simulink model "Teensy_Model"  (R2025b)
settings: Solver=FixedStepAuto  StartTime=0.0  StopTime=Inf  FixedStep=ts  RelTol=1e-3  EnableMultiTasking=on
model workspace (MAT data in the model file):
  Footcontrol = Simulink.Parameter
  Footcontrol.Value = 0
  Footcontrol.Complexity = 'real'
  Footcontrol.Dimensions = [1 1]
  Footcontrol.Description = 'Footcontrol'
  Footcontrol.DataType = 'uint8'
  GPIO_0 = Simulink.Parameter
  GPIO_0.Value = 0
  GPIO_0.Complexity = 'real'
  GPIO_0.Dimensions = [1 1]
  GPIO_0.Description = 'GPIO_0'
  GPIO_0.DataType = 'boolean'
  GPIO_1 = Simulink.Parameter
  GPIO_1.Value = 0
  GPIO_1.Complexity = 'real'
  GPIO_1.Dimensions = [1 1]
  GPIO_1.Description = 'GPIO_1'
  GPIO_1.DataType = 'boolean'
  GPIO_2 = Simulink.Parameter
  GPIO_2.Value = 0
  GPIO_2.Complexity = 'real'
  GPIO_2.Dimensions = [1 1]
  GPIO_2.Description = 'GPIO_2'
  GPIO_2.DataType = 'boolean'
  GPIO_3 = Simulink.Signal
  GPIO_3.Dimensions = -1
  GPIO_3.DimensionsMode = 'auto'
  GPIO_3.Complexity = 'real'
  GPIO_3.SampleTime = -1
  GPIO_3.SamplingMode = 'auto'
  GPIO_3.Description = 'GPIO_3'
  GPIO_3.DataType = 'uint16'
  GPIO_4 = Simulink.Signal
  GPIO_4.Dimensions = -1
  GPIO_4.DimensionsMode = 'auto'
  GPIO_4.Complexity = 'real'
  GPIO_4.SampleTime = -1
  GPIO_4.SamplingMode = 'auto'
  GPIO_4.Description = 'GPIO_4'
  GPIO_4.DataType = 'uint16'
  GPIO_5 = Simulink.Signal
  GPIO_5.Dimensions = -1
  GPIO_5.DimensionsMode = 'auto'
  GPIO_5.Complexity = 'real'
  GPIO_5.SampleTime = -1
  GPIO_5.SamplingMode = 'auto'
  GPIO_5.Description = 'GPIO_5'
  GPIO_5.DataType = 'uint16'
  MD_Current = Simulink.Signal
  MD_Current.Dimensions = -1
  MD_Current.DimensionsMode = 'auto'
  MD_Current.Complexity = 'real'
  MD_Current.SampleTime = -1
  MD_Current.SamplingMode = 'auto'
  MD_Current.Description = 'MD_Current'
  MD_Current.DataType = 'uint16'
  Motor_Enable = Simulink.Parameter
  Motor_Enable.Value = 0
  Motor_Enable.Complexity = 'real'
  Motor_Enable.Dimensions = [1 1]
  Motor_Enable.Description = 'Motor_Enable'
  Motor_Enable.DataType = 'boolean'
  Motor_Stop = Simulink.Parameter
  Motor_Stop.Value = 0
  Motor_Stop.Complexity = 'real'
  Motor_Stop.Dimensions = [1 1]
  Motor_Stop.Description = 'Motor_Stop'
  Motor_Stop.DataType = 'boolean'
  Speed_Out = Simulink.Parameter
  Speed_Out.Value = 0
  Speed_Out.Complexity = 'real'
  Speed_Out.Dimensions = [1 1]
  Speed_Out.Description = 'Speed_Out'
  Speed_Out.DataType = 'uint8'
  Status_LED = Simulink.Parameter
  Status_LED.Value = 0
  Status_LED.Complexity = 'real'
  Status_LED.Dimensions = [1 1]
  Status_LED.Description = 'Status_LED'
  Status_LED.DataType = 'boolean'
  Torq_Out = Simulink.Parameter
  Torq_Out.Value = 0
  Torq_Out.Complexity = 'real'
  Torq_Out.Dimensions = [1 1]
  Torq_Out.Description = 'Torq_Out'
  Torq_Out.DataType = 'uint8'
  Torq_Signal = Simulink.Signal
  Torq_Signal.Dimensions = -1
  Torq_Signal.DimensionsMode = 'auto'
  Torq_Signal.Complexity = 'real'
  Torq_Signal.SampleTime = -1
  Torq_Signal.SamplingMode = 'auto'
  Torq_Signal.Description = 'Torq_Signal'
  Torq_Signal.DataType = 'uint16'
  actSpeed_Motor = Simulink.Signal
  actSpeed_Motor.Dimensions = -1
  actSpeed_Motor.DimensionsMode = 'auto'
  actSpeed_Motor.Complexity = 'real'
  actSpeed_Motor.SampleTime = -1
  actSpeed_Motor.SamplingMode = 'auto'
  actSpeed_Motor.Description = 'actSpeed_Motor'
  actSpeed_Motor.DataType = 'single'
  actSpeed_Torq = Simulink.Signal
  actSpeed_Torq.Dimensions = -1
  actSpeed_Torq.DimensionsMode = 'auto'
  actSpeed_Torq.Complexity = 'real'
  actSpeed_Torq.SampleTime = -1
  actSpeed_Torq.SamplingMode = 'auto'
  actSpeed_Torq.Description = 'actSpeed_Torq'
  actSpeed_Torq.DataType = 'single'
  actTemp_48 = Simulink.Signal
  actTemp_48.Dimensions = -1
  actTemp_48.DimensionsMode = 'auto'
  actTemp_48.Complexity = 'real'
  actTemp_48.SampleTime = -1
  actTemp_48.SamplingMode = 'auto'
  actTemp_48.Description = 'actTemp_48'
  actTemp_48.DataType = 'single'
  actTemp_49 = Simulink.Signal
  actTemp_49.Dimensions = -1
  actTemp_49.DimensionsMode = 'auto'
  actTemp_49.Complexity = 'real'
  actTemp_49.SampleTime = -1
  actTemp_49.SamplingMode = 'auto'
  actTemp_49.Description = 'actTemp_49'
  actTemp_49.DataType = 'single'
values from neighbouring files (symbols this model uses):
  Footcontrol = Simulink.Parameter    [SimulinkSetup.m]
  GPIO_0 = Simulink.Parameter    [SimulinkSetup.m]
  GPIO_1 = Simulink.Parameter    [SimulinkSetup.m]
  GPIO_2 = Simulink.Parameter    [SimulinkSetup.m]
  Motor_Enable = Simulink.Parameter    [SimulinkSetup.m]
  Motor_Stop = Simulink.Parameter    [SimulinkSetup.m]
  Speed_Out = Simulink.Parameter    [SimulinkSetup.m]
  Status_LED = Simulink.Parameter    [SimulinkSetup.m]
  Torq_Out = Simulink.Parameter    [SimulinkSetup.m]
  ts = 1e-3    (= 0.001)    [SimulinkSetup.m]
libraries: arduinolib x16
settings Model: ExtModeTrigDuration=2  Creator=The MathWorks, Inc.  LastModifiedBy=Benjamin.Rutishauser
settings SolverCC: AlgebraicLoopSolver=TrustRegion  AutoInsertRateTranBlk=on  MaxZcPerStep=1.0
settings OptimizationCC: EnhancedBackFolding=on  PassReuseOutputArgsAs=Individual arguments  ZeroExternalMemoryAtStartup=off  ZeroInternalMemoryAtStartup=off  MaxStackSize=64  OptimizeBlockOrder=speed  DifferentSizesBufferReuse=on  OptimizationCustomize=off  EfficientTunableParamExpr=on
settings DebuggingCC: ParameterTunabilityLossMsg=error  UnconnectedInputMsg=warning  UnconnectedOutputMsg=warning  UnconnectedLineMsg=warning
settings HardwareCC: ProdBitPerPointer=32.0  ProdBitPerSizeT=32.0  ProdBitPerPtrDiffT=32.0  ProdLargestAtomicInteger=Long  ProdLargestAtomicFloat=Double  ProdWordSize=32.0  ProdHWDeviceType=ARM Compatible->ARM Cortex
settings ModelReferenceCC: EnableRefExpFcnMdlSchedulingChecks=on
settings SFSimCC: MATLABDynamicMemAlloc=off
settings RTWCC: SystemTargetFile=ert.tlc  HardwareBoard=Teensy 4.1 (Arduino Compatible)  TemplateMakefile=ert_default_tmf  Toolchain=Arduino ARM M7  BuildConfiguration=Faster Runs  GPUComputeCapability=3.5  DLArmComputeVersion=19.05  Description=Embedded Coder
settings CodeAppCC: ForceParamTrailComments=on  IgnoreCustomStorageClasses=off  OperatorAnnotations=on  SimulinkDataObjDesc=on  SFDataObjDesc=on  InsertBlockDesc=on
settings ERTTargetCC: ExtModeTransport=3.0  ExtModeStaticAlloc=on  ExtModeAutomaticAllocSize=off  ExtModeStaticAllocSize=65536.0  ExtModeMexFile=ext_xcp  ExtModeIntrfLevel=Level2 - Open  InlinedParameterPlacement=Hierarchical  DynamicArrayContainerType=coder::array  SupportContinuousTime=on  SupportNonInlinedSFcns=on  SupportVariableSizeSignals=on

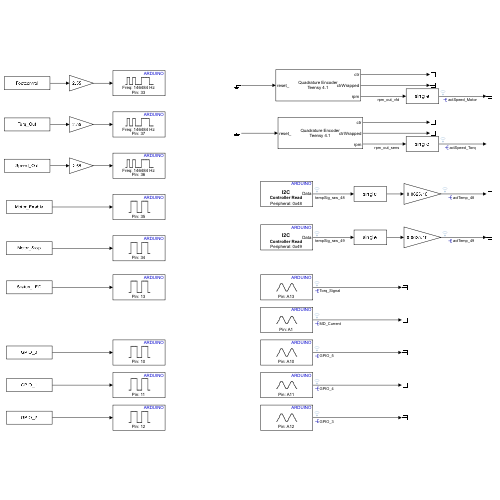
[thumbnail: Simulink's stored preview of the top-level diagram]
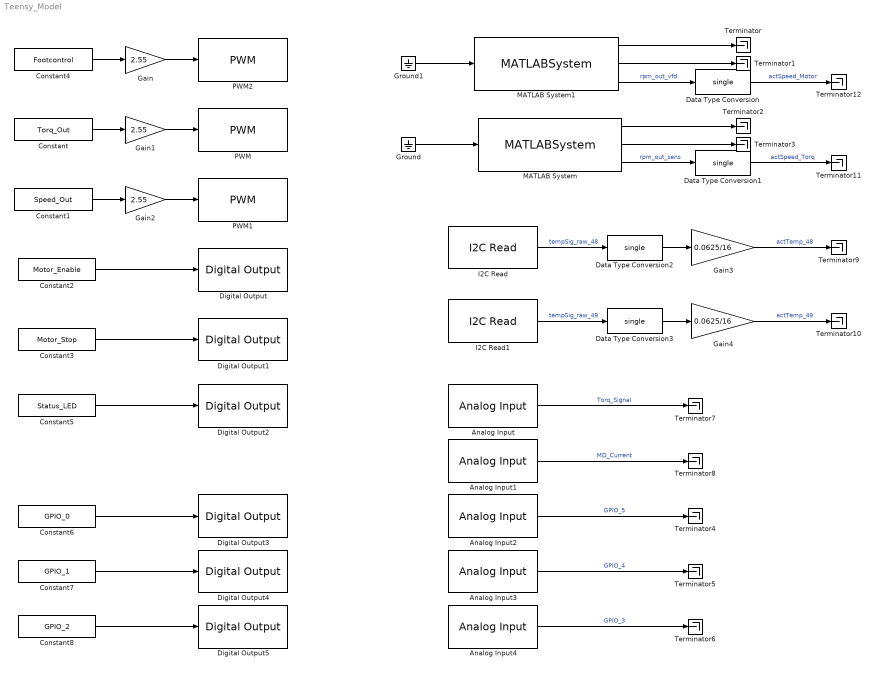
== system Teensy_Model ==
  Analog Input : arduinolib/Analog Input  pinNumber=13  ReadResultsOnly=off  ConversionTriggerSource=Software  ExternalTriggerType=uint32( 0 )  OutputDataType=uint16  EnableConversionCompleteNotify=off  EnableOuputStatus=off  SampleTime=ts  blockPlatform=arduino
      settings: LibrarySourceBlock=gizmoLibrary/Arduino Utilities/Analog Input
  Analog Input1 : arduinolib/Analog Input  pinNumber=1  ReadResultsOnly=off  ConversionTriggerSource=Software  ExternalTriggerType=uint32( 0 )  OutputDataType=uint16  EnableConversionCompleteNotify=off  EnableOuputStatus=off  SampleTime=ts  blockPlatform=arduino
      settings: LibrarySourceBlock=gizmoLibrary/Arduino Utilities/Analog Input
  Analog Input2 : arduinolib/Analog Input  pinNumber=10  ReadResultsOnly=off  ConversionTriggerSource=Software  ExternalTriggerType=uint32( 0 )  OutputDataType=uint16  EnableConversionCompleteNotify=off  EnableOuputStatus=off  SampleTime=ts  blockPlatform=arduino
  Analog Input3 : arduinolib/Analog Input  pinNumber=11  ReadResultsOnly=off  ConversionTriggerSource=Software  ExternalTriggerType=uint32( 0 )  OutputDataType=uint16  EnableConversionCompleteNotify=off  EnableOuputStatus=off  SampleTime=ts  blockPlatform=arduino
  Analog Input4 : arduinolib/Analog Input  pinNumber=12  ReadResultsOnly=off  ConversionTriggerSource=Software  ExternalTriggerType=uint32( 0 )  OutputDataType=uint16  EnableConversionCompleteNotify=off  EnableOuputStatus=off  SampleTime=ts  blockPlatform=arduino
  Constant : Constant  Value=Torq_Out
  Constant1 : Constant  Value=Speed_Out
  Constant2 : Constant  Value=Motor_Enable
  Constant3 : Constant  Value=Motor_Stop
  Constant4 : Constant  Value=Footcontrol
  Constant5 : Constant  Value=Status_LED
  Constant6 : Constant  Value=GPIO_0
  Constant7 : Constant  Value=GPIO_1
  Constant8 : Constant  Value=GPIO_2
  Data Type Conversion{,1..3} (4 alike) : DataTypeConversion  OutDataTypeStr=single  SaturateOnIntegerOverflow=off  RndMeth=Floor
  Digital Output : arduinolib/Digital Output  pinNumber=35  Direction=output  blockPlatform=arduino
  Digital Output1 : arduinolib/Digital Output  pinNumber=34  Direction=output  blockPlatform=arduino
  Digital Output2 : arduinolib/Digital Output  pinNumber=13  Direction=output  blockPlatform=arduino
  Digital Output3 : arduinolib/Digital Output  pinNumber=10  Direction=output  blockPlatform=arduino
  Digital Output4 : arduinolib/Digital Output  pinNumber=11  Direction=output  blockPlatform=arduino
  Digital Output5 : arduinolib/Digital Output  pinNumber=12  Direction=output  blockPlatform=arduino
  Gain : Gain  Gain=2.55  OutDataTypeStr=double
  Gain1 : Gain  Gain=2.55  OutDataTypeStr=double
  Gain2 : Gain  Gain=2.55  OutDataTypeStr=double
  Gain3 : Gain  Gain=0.0625/16
  Gain4 : Gain  Gain=0.0625/16
  Ground : Ground
  Ground1 : Ground
  I2C Read : arduinolib/I2C Read  I2CModule=0  Mode=Master  SlaveAddress=0x48  SlaveByteOrder=BigEndian  Direction=Receiver  RegisterAddressMode=on  RegisterAddress=0x00  SlaveDataType=uint16  DataLength=1  NoAck=off  RepeatedStart=off  OutputStatus=off  blockPlatform=ARDUINO  SampleTime=0.25
  I2C Read1 : arduinolib/I2C Read  I2CModule=0  Mode=Master  SlaveAddress=0x49  SlaveByteOrder=BigEndian  Direction=Receiver  RegisterAddressMode=on  RegisterAddress=0x00  SlaveDataType=uint16  DataLength=1  NoAck=off  RepeatedStart=off  OutputStatus=off  blockPlatform=ARDUINO  SampleTime=0.25
  MATLAB System : MATLABSystem  System=QuadEncTeensy  encChannel=uint8(1)  phaseA=uint8(3)  phaseB=uint8(4)  res=360*4  ts=ts  filterN=20
      mask Type: QuadEncTeensy
  MATLAB System1 : MATLABSystem  System=QuadEncTeensy  encChannel=uint8(2)  phaseA=uint8(2)  phaseB=uint8(8)  res=2 ^ 11 * 4  ts=ts  filterN=30
      mask Type: QuadEncTeensy
  PWM : arduinolib/PWM  pinNumber=37  frequencyType=Specify  desiredFrequency=pwmFreq  achievableFrequency=146484
  PWM1 : arduinolib/PWM  pinNumber=36  frequencyType=Specify  desiredFrequency=pwmFreq  achievableFrequency=146484
  PWM2 : arduinolib/PWM  pinNumber=33  frequencyType=Specify  desiredFrequency=pwmFreq  achievableFrequency=146484
  Terminator{,1..12} (13 alike) : Terminator
  wires:
  Data Type Conversion/1 -> Terminator12/1  "actSpeed_Motor"
  Data Type Conversion1/1 -> Terminator11/1  "actSpeed_Torq"
  Ground/1 -> MATLAB System/1
  Ground1/1 -> MATLAB System1/1
  MATLAB System1/1 -> Terminator/1
  MATLAB System1/2 -> Terminator1/1
  MATLAB System/2 -> Terminator3/1
  MATLAB System/1 -> Terminator2/1
  Constant/1 -> Gain1/1
  Constant1/1 -> Gain2/1
  Constant2/1 -> Digital Output/1
  Constant3/1 -> Digital Output1/1
  Constant4/1 -> Gain/1
  Gain/1 -> PWM2/1
  Gain1/1 -> PWM/1
  Gain2/1 -> PWM1/1
  Analog Input/1 -> Terminator7/1  "Torq_Signal"
  Analog Input1/1 -> Terminator8/1  "MD_Current"
  Constant5/1 -> Digital Output2/1
  MATLAB System1/3 -> Data Type Conversion/1  "rpm_out_vfd"
  MATLAB System/3 -> Data Type Conversion1/1  "rpm_out_sens"
  Gain3/1 -> Terminator9/1  "actTemp_48"
  Data Type Conversion2/1 -> Gain3/1
  I2C Read/1 -> Data Type Conversion2/1  "tempSig_raw_48"
  Gain4/1 -> Terminator10/1  "actTemp_49"
  Data Type Conversion3/1 -> Gain4/1
  I2C Read1/1 -> Data Type Conversion3/1  "tempSig_raw_49"
  Constant6/1 -> Digital Output3/1
  Constant7/1 -> Digital Output4/1
  Constant8/1 -> Digital Output5/1
  Analog Input2/1 -> Terminator4/1  "GPIO_5"
  Analog Input3/1 -> Terminator5/1  "GPIO_4"
  Analog Input4/1 -> Terminator6/1  "GPIO_3"
